simulink model "aula_ca_11_12_23"  (R2022a)
settings: Solver=VariableStepAuto  StartTime=0.0  StopTime=40  RelTol=1e-3
settings Model: Creator=Aluno  LastModifiedBy=Aluno

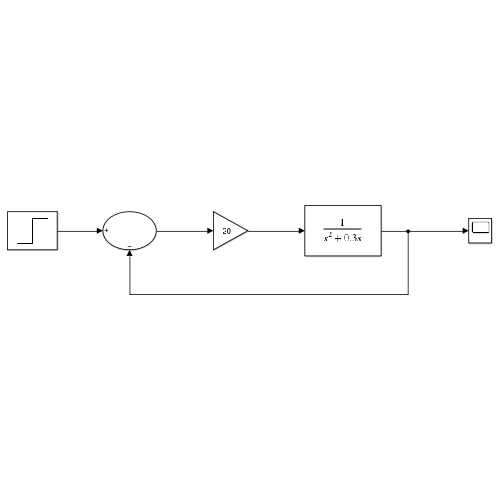
[thumbnail: Simulink's stored preview of the top-level diagram]
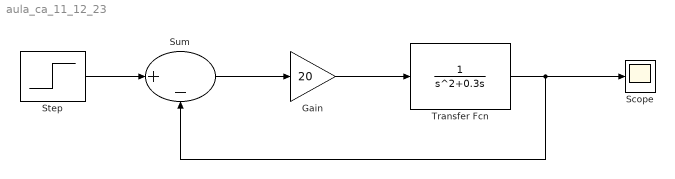
== system aula_ca_11_12_23 ==
  Gain : Gain  Gain=20
  Scope : Scope
  Step : Step  Time=0  SampleTime=0
  Sum : Sum  Inputs=|+-
  Transfer Fcn : TransferFcn  Denominator=[1 0.3 0]
  wires:
  Step/1 -> Sum/1
  Sum/1 -> Gain/1
  Gain/1 -> Transfer Fcn/1
  Transfer Fcn/1 -> Sum/2, Scope/1
